simulink model "sim3d_14DoF_visualization"  (R2024b)
settings: Solver=VariableStepAuto  StartTime=0.0  StopTime=10.0  RelTol=1e-3
undefined symbols (not defined in the file or in its folder): sampleScene, simple_straight_unEven
libraries: sim3dlib x3, simulink x2, sim3dautolib x1
settings Model: Creator=fukuchi  LastModifiedBy=nobuakif

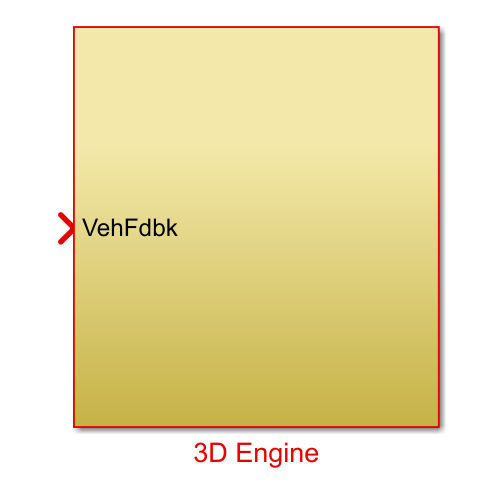
[thumbnail: Simulink's stored preview of the top-level diagram]
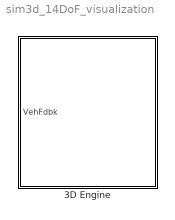
== system sim3d_14DoF_visualization ==
  3D Engine : Subsystem  VariantControl=engine3D==1

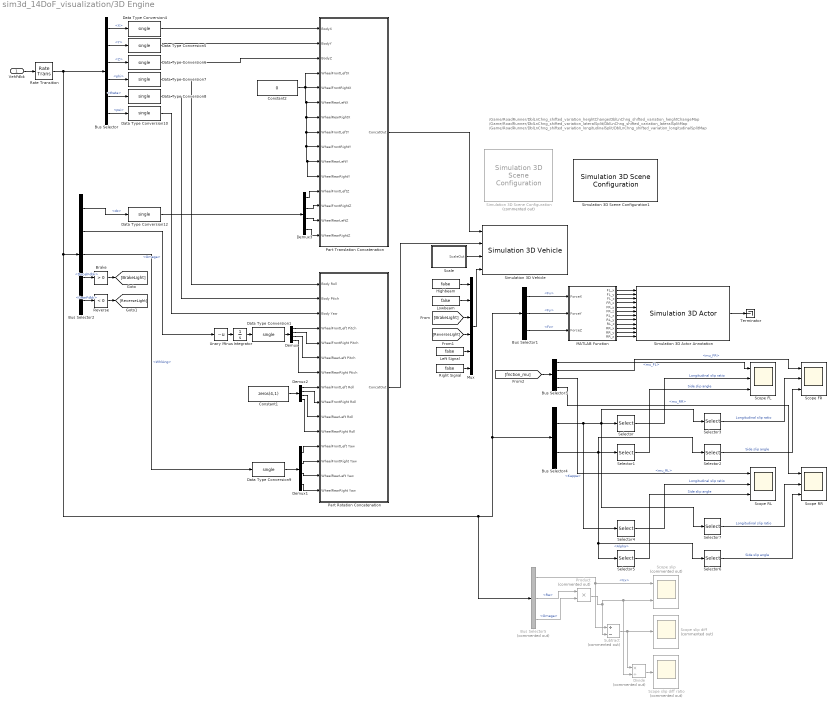
== system sim3d_14DoF_visualization/3D Engine ==
  note: /Game/RoadRunner/DblLnChng_shifted_variation_heightChange/DblLnChng_shifted_variation_heightChangeMap
      | /Game/RoadRunner/DblLnChng_shifted_variation_lateralSplit/DblLnChng_shifted_variation_lateralSplitMap
      | /Game/RoadRunner/DblLnChng_shifted_variation_longitudinalSplit/DblLnChng_shifted_variation_longitudinalSplitMap
  VehFdbk : Inport
  Brake : simulink/Logic and Bit Operations/Compare To Constant  relop=>  const=0  OutDataTypeStr=boolean  ZeroCross=off
  Bus Selector : BusSelector  OutputSignals=Body.InertFrm.Geom.Disp.X,Body.InertFrm.Geom.Disp.Y,Body.InertFrm.Geom.Disp.Z,Body.InertFrm.Cg.Ang.phi,Body.InertFrm.Cg.Ang.theta,Body.InertFrm.Cg.Ang.psi
  Bus Selector1 : BusSelector  OutputSignals=Wheels.TireFrame.Fx,Wheels.TireFrame.Fy,Wheels.TireFrame.Fz
  Bus Selector2 : BusSelector  OutputSignals=Wheels.TireFrame.dz,Wheels.TireFrame.Omega,Driveline.WhlAng,Driver.DecelFdbk,Driver.GearFdbk
  Bus Selector3 : BusSelector  OutputSignals=mu_FL,mu_FR,mu_RL,mu_RR
  Bus Selector4 : BusSelector  OutputSignals=Wheels.TireFrame.Kappa,Wheels.TireFrame.Alpha
  Bus Selector5 : BusSelector  Commented=on  OutputSignals=Wheels.TireFrame.Vx,Wheels.TireFrame.Re,Wheels.TireFrame.Omega
  Constant1 : Constant  Value=zeros(4,1)  OutDataTypeStr=single
  Constant2 : Constant  Value=0  OutDataTypeStr=single
  Data Type Conversion{1,4..10,12} (9 alike) : DataTypeConversion  OutDataTypeStr=single  SaturateOnIntegerOverflow=off  RndMeth=Floor
  Demux{,1..3} (4 alike) : Demux
  Divide : Product  Commented=on  Inputs=*/
  Highbeam : Constant  Value=false
  Integrator : Integrator  WrapState=on  WrappedStateUpperValue=2*pi  WrappedStateLowerValue=0  ZeroCross=off
  Left Signal : Constant  Value=false
  Lowbeam : Constant  Value=false
  MATLAB Function : MATLAB Function  TreatAsAtomicUnit=on
  Mux : Mux  Inputs=6
  Part Rotation Concatenation : Subsystem
  Part Translation Concatenation : Subsystem
  Product : Product  Commented=on
  Rate Transition : RateTransition  OutPortSampleTime=0.1
  Reverse : simulink/Logic and Bit Operations/Compare To Constant  relop=<  const=0  OutDataTypeStr=boolean  ZeroCross=off
  Right Signal : Constant  Value=false
  Scale : Subsystem
  Scope FL : Scope  NumInputPorts=3
  Scope FR : Scope  NumInputPorts=3
  Scope RL : Scope  NumInputPorts=3
  Scope RR : Scope  NumInputPorts=3
  Scope slip : Scope  Commented=on  NumInputPorts=2
  Scope slip diff : Scope  Commented=on
  Scope slip diff ratio : Scope  Commented=on
  Selector : Selector  InputPortWidth=4  IndexOptions=Index vector (dialog)  Indices=1  OutputSizes=1
  Selector1 : Selector  InputPortWidth=4  IndexOptions=Index vector (dialog)  Indices=1  OutputSizes=1
  Selector2 : Selector  InputPortWidth=4  IndexOptions=Index vector (dialog)  Indices=2  OutputSizes=1
  Selector3 : Selector  InputPortWidth=4  IndexOptions=Index vector (dialog)  Indices=2  OutputSizes=1
  Selector4 : Selector  InputPortWidth=4  IndexOptions=Index vector (dialog)  Indices=3  OutputSizes=1
  Selector5 : Selector  InputPortWidth=4  IndexOptions=Index vector (dialog)  Indices=3  OutputSizes=1
  Selector6 : Selector  InputPortWidth=4  IndexOptions=Index vector (dialog)  Indices=4  OutputSizes=1
  Selector7 : Selector  InputPortWidth=4  IndexOptions=Index vector (dialog)  Indices=4  OutputSizes=1
  Simulation 3D Actor Annotation : sim3dlib/Simulation 3D Actor  Priority=1  ActorName=Sim3dActor_annotation  ParentName=SimulinkVehicle1  Operation=Create at setup  InitScriptText=|  SampleTime=-1  Translation=single([0 0 0])  Rotation=single([0 0 0])  Scale=single([1 1 1])  InputsText=|  aMode=5  ActorTag=Sim3dActor_annotation  ActorType=Sim3dActor  ID=C
      InitScriptText=|
      | y_offset = 1; z_offset = 0.1;
      | fl_pos = [1.491, 1.713/2+y_offset, z_offset];
      | fr_pos = [1.491, -1.713/2-y_offset, z_offset];
      | rl_pos = [-1.592, 1.713/2+y_offset, z_offset];
      | rr_pos = [-1.592, -1.713/2-y_offset, z_offset];
      | 
      | arrowfl = sim3d.graphics.Arrow("ActorName", "FL_Z");
      | arrowfl.CoordinateSystem = "MATLAB";
      | arrowfl.Color = [0, 0, 1];
      | arrowfl.Rotation = [0, -pi/2, 0];
      | arrowfl.Scale = [1, 1, 1]*2;
      | World.add(arrowfl, Actor);
      | arrowfl.Translation = fl_pos;
      | 
      | arrowfl_x = sim3d.graphics.Arrow("ActorName", "FL_X");
      | arrowfl_x.CoordinateSystem = "MATLAB";
      | arrowfl_x.Color = [1, 0, 0];
      | arrowfl_x.Rotation = [0, 0, 0];
      | arrowfl_x.Scale = [1, 1, 1]*2;
      | World.add(arrowfl_x, Actor);
      | arrowfl_x.Translation = fl_pos;
      | 
      | arrowfl_y = sim3d.graphics.Arrow("ActorName", "FL_Y");
      | arrowfl_y.CoordinateSystem = "MATLAB";
      | arrowfl_y.Color = [0, 1, 0];
      | arrowfl_y.Rotation = [0, 0, pi/2];
      | arrowfl_y.Scale = [1, 1, 1]*2;
      | World.add(arrowfl_y, Actor);
      | arrowfl_y.Translation = fl_pos;
      | 
      | 
      | arrowfr = sim3d.graphics.Arrow("ActorName", "FR_Z");
      | arrowfr.CoordinateSystem = "MATLAB";
      | arrowfr.Color = [0, 0, 1];
      | arrowfr.Rotation = [0, -pi/2, 0];
      | arrowfr.Scale = [1, 1, 1] * 2;
      | World.add(arrowfr, Actor);
      | arrowfr.Translation = fr_pos;
      | 
      | arrowfr_x = sim3d.graphics.Arrow("ActorName", "FR_X");
      | arrowfr_x.CoordinateSystem = "MATLAB";
      | arrowfr_x.Color = [1, 0, 0];
      | arrowfr_x.Rotation = [0, 0, 0];
      | arrowfr_x.Scale = [1, 1, 1]*2;
      | World.add(arrowfr_x, Actor);
      | arrowfr_x.Translation = fr_pos;
      | 
      | arrowfr_y = sim3d.graphics.Arrow("ActorName", "FR_Y");
      | arrowfr_y.CoordinateSystem = "MATLAB";
      | arrowfr_y.Color = [0, 1, 0];
      | arrowfr_y.Rotation = [0, 0, pi/2];
      | arrowfr_y.Scale = [1, 1, 1]*2;
      | World.add(arrowfr_y, Actor);
      | arrowfr_y.Translation = fr_pos;
      | 
      | 
      | arrowrl = sim3d.graphics.Arrow("ActorName", "RL_Z");
      | arrowrl.CoordinateSystem = "MATLAB";
      | arrowrl.Color = [0, 0, 1];
      | arrowrl.Rotation = [0, -pi/2, 0];
      | arrowrl.Scale = [1, 1, 1] * 2;
      | World.add(arrowrl, Actor);
      | arrowrl.Translation = rl_pos;
      | 
      | arrowrl_x = sim3d.graphics.Arrow("ActorName", "RL_X");
      | arrowrl_x.CoordinateSystem = "MATLAB";
      | arrowrl_x.Color = [1, 0, 0];
      | arrowrl_x.Rotation = [0, 0, 0];
      | arrowrl_x.Scale = [1, 1, 1]*2;
      | World.add(arrowrl_x, Actor);
      | arrowrl_x.Translation = rl_pos;
      | 
      | arrowrl_y = sim3d.graphics.Arrow("ActorName", "RL_Y");
      | arrowrl_y.CoordinateSystem = "MATLAB";
      | arrowrl_y.Color = [0, 1, 0];
      | arrowrl_y.Rotation = [0, 0, pi/2];
      | arrowrl_y.Scale = [1, 1, 1]*2;
      | World.add(arrowrl_y, Actor);
      | arrowrl_y.Translation = rl_pos;
      | 
      | 
      | arrowrr = sim3d.graphics.Arrow("ActorName", "RR_Z");
      | arrowrr.CoordinateSystem = "MATLAB";
      | arrowrr.Color = [0, 0, 1];
      | arrowrr.Rotation = [0, -pi/2, 0];
      | arrowrr.Scale = [1, 1, 1]*2;
      | World.add(arrowrr, Actor);
      | arrowrr.Translation = rr_pos;
      | 
      | arrowrr_x = sim3d.graphics.Arrow("ActorName", "RR_X");
      | arrowrr_x.CoordinateSystem = "MATLAB";
      | arrowrr_x.Color = [1, 0, 0];
      | arrowrr_x.Rotation = [0, 0, 0];
      | arrowrr_x.Scale = [1, 1, 1]*2;
      | World.add(arrowrr_x, Actor);
      | arrowrr_x.Translation = rr_pos;
      | 
      | arrowrr_y = sim3d.graphics.Arrow("ActorName", "RR_Y");
      | arrowrr_y.CoordinateSystem = "MATLAB";
      | arrowrr_y.Color = [0, 1, 0];
      | arrowrr_y.Rotation = [0, 0, pi/2];
      | arrowrr_y.Scale = [1, 1, 1]*2;
      | World.add(arrowrr_y, Actor);
      | arrowrr_y.Translation = rr_pos;
      InputsText=|
      | FL_X.Scale
      | FL_Y.Scale
      | FL_Z.Scale
      | FR_X.Scale
      | FR_Y.Scale
      | FR_Z.Scale
      | RL_X.Scale
      | RL_Y.Scale
      | RL_Z.Scale
      | RR_X.Scale
      | RR_Y.Scale
      | RR_Z.Scale
  Simulation 3D Scene Configuration : sim3dlib/Simulation 3D Scene Configuration  Priority=0  Commented=on  ProjectFormat=RoadRunner  SceneDesc=Double lane change  ProjectName=D:\MATLAB\R2024b\toolbox\shared\sim3d_projects\automotive_project_windows\UE\WindowsNoEditor\VehicleSimulation.exe  ScenePath=/Game/RoadRunner/DblLnChng_shifted_variation_longitudinalSplit/DblLnChng_shifted_variation_longitudinalSplitMap  RoadRunnerProjectPath=sampleScene/simple_straight_unEven.fbx  UEProjPath=D:\ADT_UE4\R2024aGR\AutoVrtlEnv\AutoVrtlEnv.uproject  EnableOpenDRIVE=off  vehTagList={'Custom';'Scene Origin';'Sim3dActor_annotation';'SimulinkVehicle1'}  vehTag=Sim3dActor_annotation  FreeCameraInitialTranslation=[0, 0, 0]  FreeCameraDefaultInitialTranslation=[-6, 0, 2]  FreeCameraInitialRotation=[0, 0, 0]  FreeCameraDefaultInitialRotation=[0, -15, 0]  OpVisEn=off  Ts=0.1  EnableWindow=on  EnableRemoteAccess=off  EnableWeather=off  SunAzimuth=90  SunAltitude=40.0  EnableGeospatialSun=off  Latitude=0  Longitude=0  Date=2023-01-01  Time=10:30:00  GeoTimeZone=-5.0  SunDaylightSaving=off  wind=1  clouds=10  EnableVolumetricClouds=off  CloudCoverage=0  CloudAltitude=6  fog=0  rain=0  RaindropsEffect=off  SnowDensity=0  EnableGeospatial=off  UseTrueOrigin=off  OriginHeight=200  OriginLatitude=40.744652  OriginLongitude=-73.988864  MapStyle=Aerial  AdditionalAssetIDs=[]  UseAdvancedSunSky=off  SolarTime=11  TimeZone=-5  Day=21  Month=9  Year=2022  UseDaylightSavingTime=on  DSTStartDay=10  DSTStartMonth=3  DSTEndDay=3  DSTEndMonth=11  DSTSwitchHour=2  sensorTag=MainCamera1  sensorId=1  sensorName=MainCamera1  mountLoc=Origin  offsetFlag=off  tmountOffset=[0, 0, 0]  rmountOffset=[0, 0, 0]  HorizontalResolution=1280  VerticalResolution=720  HorizontalFOV=60  mountPoint=[0 0 0]  mountOrientation=[0 0 0]  aMode=2  ID=1  GeoTrigger=Inactive
      settings: LibrarySourceBlock=vehdynlibsim3dcore/Simulation 3D Scene Configuration
  Simulation 3D Scene Configuration1 : sim3dlib/Simulation 3D Scene Configuration  Priority=0  ProjectFormat=Default Scenes  SceneDesc=Empty scene  ProjectName=D:\MATLAB\R2024b\toolbox\shared\sim3d_projects\automotive_project_windows\UE\WindowsNoEditor\VehicleSimulation.exe  ScenePath=/Game/Maps/HwStrght  EnableOpenDRIVE=off  vehTagList={'Custom';'Scene Origin';'Sim3dActor_annotation';'SimulinkVehicle1'}  vehTag=SimulinkVehicle1  FreeCameraInitialTranslation=[0, 0, 0]  FreeCameraDefaultInitialTranslation=[-6, 0, 2]  FreeCameraInitialRotation=[0, 0, 0]  FreeCameraDefaultInitialRotation=[0, -15, 0]  OpVisEn=off  Ts=0.1  EnableWindow=on  EnableRemoteAccess=off  EnableWeather=off  SunAzimuth=90  SunAltitude=40.0  EnableGeospatialSun=off  Latitude=0  Longitude=0  Date=2023-01-01  Time=10:30:00  GeoTimeZone=-5.0  SunDaylightSaving=off  wind=1  clouds=10  EnableVolumetricClouds=off  CloudCoverage=0  CloudAltitude=6  fog=0  rain=0  RaindropsEffect=off  SnowDensity=0  EnableGeospatial=off  UseTrueOrigin=off  OriginHeight=200  OriginLatitude=40.744652  OriginLongitude=-73.988864  MapStyle=Aerial  AdditionalAssetIDs=[]  UseAdvancedSunSky=off  SolarTime=11  TimeZone=-5  Day=21  Month=9  Year=2022  UseDaylightSavingTime=on  DSTStartDay=10  DSTStartMonth=3  DSTEndDay=3  DSTEndMonth=11  DSTSwitchHour=2  sensorTag=MainCamera2  sensorId=2  sensorName=MainCamera2  mountLoc=Origin  offsetFlag=off  tmountOffset=[0, 0, 0]  rmountOffset=[0, 0, 0]  HorizontalResolution=1280  VerticalResolution=720  HorizontalFOV=60  mountPoint=[0 0 0]  mountOrientation=[0 0 0]  aMode=5  ID=2  GeoTrigger=Inactive
      settings: LibrarySourceBlock=sl3dlib/Simulation 3D/Environment/Simulation 3D Scene Configuration
  Simulation 3D Vehicle : sim3dautolib/Simulation 3D Vehicle  Priority=-1  PassVehMesh=Muscle car  MeshPath=/MathWorksSimulation/Vehicles/Muscle/Meshes/SK_MuscleCar.SK_MuscleCar  VehColor=Red  ActorName=SimulinkVehicle1  VehLightsControl=on  HeadlightColor=[ 1, 1, 1 ]  HighBeamIntensity=100000  LowBeamIntensity=60000  HighBeamConeAngle=1.22  LowBeamConeAngle=1.22  LeftHeadlightOrientation=[ 0, 0 ]  RightHeadlightOrientation=[ 0, 0 ]  BrakelightIntensity=500  ReverselightIntensity=500  SignallightIntensity=500  SignallightPeriod=1  SignalPulseWidth=50  Translation=zeros(5,3)  Rotation=zeros(5,3)  Scale=ones( 5, 3 )  SampleTime=-1  ActorType=SimulinkVehicle  ID=1  aMode=2  ActorTag=SimulinkVehicle1
  Subtract : Sum  Commented=on  Inputs=+-
  Terminator : Terminator
  Unary Minus : UnaryMinus
  wires:
  Unary Minus/1 -> Integrator/1
  Bus Selector2/1 -> Data Type Conversion12/1  "<dz>"
  Rate Transition/1 -> Bus Selector/1, Bus Selector2/1, Bus Selector5/1, Bus Selector1/1, Bus Selector4/1
  Scale/1(ScaleOut) -> Simulation 3D Vehicle/3
  Demux/4 -> Part Rotation Concatenation/7(WheelRearRight Ptich)
  Demux/3 -> Part Rotation Concatenation/6(WheelRearLeft Pitch)
  Demux/2 -> Part Rotation Concatenation/5(WheelFrontRight Pitch)
  Demux/1 -> Part Rotation Concatenation/4(WheelFrontLeft Pitch)
  Constant1/1 -> Demux2/1
  Bus Selector/4 -> Data Type Conversion7/1  "<phi>"
  Part Rotation Concatenation/1(ConcatOut) -> Simulation 3D Vehicle/2
  Part Translation Concatenation/1(ConcatOut) -> Simulation 3D Vehicle/1
  Data Type Conversion12/1 -> Demux3/1
  Demux3/4 -> Part Translation Concatenation/15(WheelRearRightZ)
  Demux3/3 -> Part Translation Concatenation/14(WheelRearLeftZ)
  Demux3/1 -> Part Translation Concatenation/12(WheelFrontLeftZ)
  Demux3/2 -> Part Translation Concatenation/13(WheelFrontRightZ)
  VehFdbk/1 -> Rate Transition/1
  Data Type Conversion6/1 -> Part Translation Concatenation/3(BodyZ)
  Demux1/4 -> Part Rotation Concatenation/15(WheelRearRight Yaw)
  Demux1/3 -> Part Rotation Concatenation/14(WheelRearLeft Yaw)
  Demux2/1 -> Part Rotation Concatenation/8(WheelFrontLeft Roll)
  Demux2/2 -> Part Rotation Concatenation/9(WheelFrontRight Roll)
  Demux2/3 -> Part Rotation Concatenation/10(WheelRearLeft Roll)
  Demux2/4 -> Part Rotation Concatenation/11(WheelRearRight Roll)
  Bus Selector2/3 -> Data Type Conversion9/1  "<WhlAng>"
  Bus Selector2/2 -> Unary Minus/1  "<Omega>"
  Data Type Conversion9/1 -> Demux1/1
  Demux1/1 -> Part Rotation Concatenation/12(WheelFrontLeft Yaw)
  Demux1/2 -> Part Rotation Concatenation/13(WheelFrontRight Yaw)
  Integrator/1 -> Data Type Conversion1/1
  Data Type Conversion1/1 -> Demux/1
  Data Type Conversion8/1 -> Part Rotation Concatenation/2(Body Ptich)
  Data Type Conversion5/1 -> Part Translation Concatenation/2(BodyY)
  Data Type Conversion10/1 -> Part Rotation Concatenation/3(Body Yaw)
  Constant2/1 -> Part Translation Concatenation/5(WheelFrontRightX), Part Translation Concatenation/6(WheelRearLeftX), Part Translation Concatenation/7(WheelRearRightX), Part Translation Concatenation/8(WheelFrontLeftY), Part Translation Concatenation/9(WheelFrontRightY), Part Translation Concatenation/10(WheelRearLeftY), Part Translation Concatenation/11(WheelRearRightY), Part Translation Concatenation/4(WheelFrontLeftX)
  Data Type Conversion4/1 -> Part Translation Concatenation/1(BodyX)
  Data Type Conversion7/1 -> Part Rotation Concatenation/1(Body Roll)
  Bus Selector/1 -> Data Type Conversion4/1  "<X>"
  Bus Selector/2 -> Data Type Conversion5/1  "<Y>"
  Bus Selector/3 -> Data Type Conversion6/1  "<Z>"
  Bus Selector/6 -> Data Type Conversion10/1  "<psi>"
  Bus Selector/5 -> Data Type Conversion8/1  "<theta>"
  [BrakeLight] -> Mux/3
  Mux/1 -> Simulation 3D Vehicle/4
  Brake/1 -> [BrakeLight]
  Highbeam/1 -> Mux/1
  Reverse/1 -> [ReverseLight]
  [ReverseLight] -> Mux/4
  Lowbeam/1 -> Mux/2
  Right Signal/1 -> Mux/6
  Left Signal/1 -> Mux/5
  Bus Selector2/4 -> Brake/1  "<DecelFdbk>"
  Bus Selector2/5 -> Reverse/1  "<GearFdbk>"
  Bus Selector1/1 -> MATLAB Function/1(ForceX)  "<Fx>"
  Bus Selector1/2 -> MATLAB Function/2(ForceY)  "<Fy>"
  Bus Selector1/3 -> MATLAB Function/3(ForceZ)  "<Fz>"
  MATLAB Function/1(FL_x) -> Simulation 3D Actor Annotation/1
  MATLAB Function/2(FL_y) -> Simulation 3D Actor Annotation/2
  MATLAB Function/3(FL_z) -> Simulation 3D Actor Annotation/3
  MATLAB Function/4(FR_x) -> Simulation 3D Actor Annotation/4
  MATLAB Function/5(FR_y) -> Simulation 3D Actor Annotation/5
  MATLAB Function/6(FR_z) -> Simulation 3D Actor Annotation/6
  MATLAB Function/7(RL_x) -> Simulation 3D Actor Annotation/7
  MATLAB Function/8(RL_y) -> Simulation 3D Actor Annotation/8
  MATLAB Function/9(RL_z) -> Simulation 3D Actor Annotation/9
  MATLAB Function/10(RR_x) -> Simulation 3D Actor Annotation/10
  MATLAB Function/11(RR_y) -> Simulation 3D Actor Annotation/11
  MATLAB Function/12(RR_z) -> Simulation 3D Actor Annotation/12
  [friction_mu] -> Bus Selector3/1
  Bus Selector3/1 -> Scope FL/1  "<mu_FL>"
  Selector/1 -> Scope FL/2  "Longitudinal slip ratio"
  Selector1/1 -> Scope FL/3  "Side slip angle"
  Bus Selector3/2 -> Scope FR/1  "<mu_FR>"
  Selector3/1 -> Scope FR/2  "Longitudinal slip ratio"
  Selector2/1 -> Scope FR/3  "Side slip angle"
  Selector6/1 -> Scope RR/3  "Side slip angle"
  Selector7/1 -> Scope RR/2  "Longitudinal slip ratio"
  Selector5/1 -> Scope RL/3  "Side slip angle"
  Selector4/1 -> Scope RL/2  "Longitudinal slip ratio"
  Bus Selector4/2 -> Selector5/1, Selector6/1, Selector2/1, Selector1/1  "<Alpha>"
  Bus Selector4/1 -> Selector4/1, Selector7/1, Selector3/1, Selector/1  "<Kappa>"
  Bus Selector3/3 -> Scope RL/1  "<mu_RL>"
  Bus Selector3/4 -> Scope RR/1  "<mu_RR>"
  Simulation 3D Actor Annotation/1 -> Terminator/1
  Bus Selector5/1 -> Subtract/1, Scope slip/1  "<Vx>"
  Bus Selector5/2 -> Product/1  "<Re>"
  Bus Selector5/3 -> Product/2  "<Omega>"
  Product/1 -> Subtract/2, Divide/2, Scope slip/2
  Subtract/1 -> Divide/1, Scope slip diff/1
  Divide/1 -> Scope slip diff ratio/1

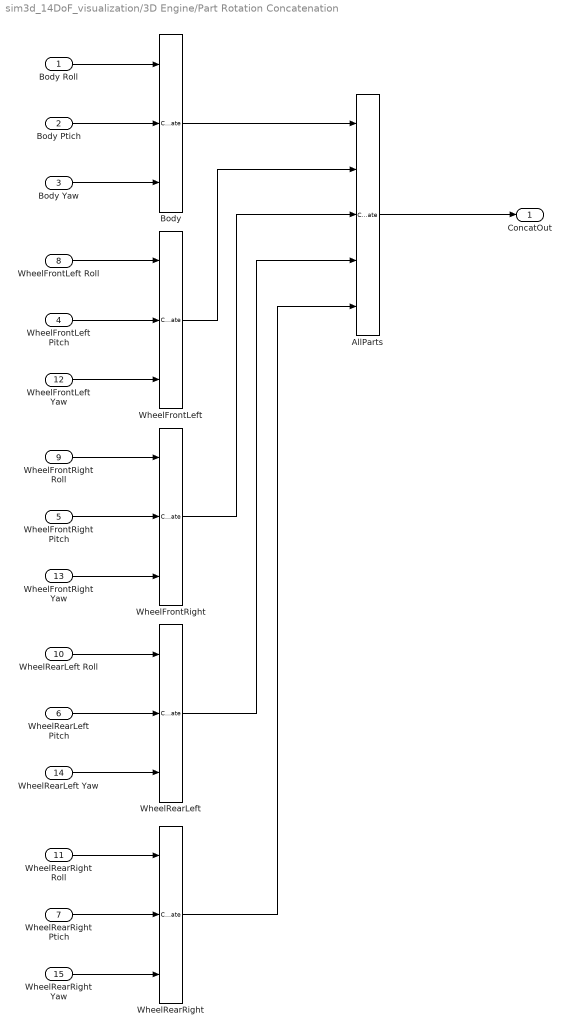
== system sim3d_14DoF_visualization/3D Engine/Part Rotation Concatenation ==
  Body Roll : Inport
  Body Ptich : Inport  Port=2
  Body Yaw : Inport  Port=3
  WheelFrontLeft Pitch : Inport  Port=4
  WheelFrontRight Pitch : Inport  Port=5
  WheelRearLeft Pitch : Inport  Port=6
  WheelRearRight Ptich : Inport  Port=7
  WheelFrontLeft Roll : Inport  Port=8
  WheelFrontRight Roll : Inport  Port=9
  WheelRearLeft Roll : Inport  Port=10
  WheelRearRight Roll : Inport  Port=11
  WheelFrontLeft Yaw : Inport  Port=12
  WheelFrontRight Yaw : Inport  Port=13
  WheelRearLeft Yaw : Inport  Port=14
  WheelRearRight Yaw : Inport  Port=15
  AllParts : Concatenate  NumInputs=5  Mode=Multidimensional array
  Body : Concatenate  NumInputs=3  Mode=Multidimensional array  ConcatenateDimension=2
  WheelFrontLeft : Concatenate  NumInputs=3  Mode=Multidimensional array  ConcatenateDimension=2
  WheelFrontRight : Concatenate  NumInputs=3  Mode=Multidimensional array  ConcatenateDimension=2
  WheelRearLeft : Concatenate  NumInputs=3  Mode=Multidimensional array  ConcatenateDimension=2
  WheelRearRight : Concatenate  NumInputs=3  Mode=Multidimensional array  ConcatenateDimension=2
  ConcatOut : Outport  VectorParamsAs1DForOutWhenUnconnected=off
  wires:
  Body Yaw/1 -> Body/3
  WheelFrontLeft Yaw/1 -> WheelFrontLeft/3
  WheelFrontLeft/1 -> AllParts/2
  Body/1 -> AllParts/1
  WheelRearLeft/1 -> AllParts/4
  WheelFrontRight/1 -> AllParts/3
  WheelRearRight Yaw/1 -> WheelRearRight/3
  WheelRearLeft Yaw/1 -> WheelRearLeft/3
  AllParts/1 -> ConcatOut/1
  WheelRearRight/1 -> AllParts/5
  WheelFrontRight Yaw/1 -> WheelFrontRight/3
  Body Roll/1 -> Body/1
  Body Ptich/1 -> Body/2
  WheelFrontLeft Pitch/1 -> WheelFrontLeft/2
  WheelFrontLeft Roll/1 -> WheelFrontLeft/1
  WheelFrontRight Roll/1 -> WheelFrontRight/1
  WheelFrontRight Pitch/1 -> WheelFrontRight/2
  WheelRearLeft Roll/1 -> WheelRearLeft/1
  WheelRearLeft Pitch/1 -> WheelRearLeft/2
  WheelRearRight Roll/1 -> WheelRearRight/1
  WheelRearRight Ptich/1 -> WheelRearRight/2

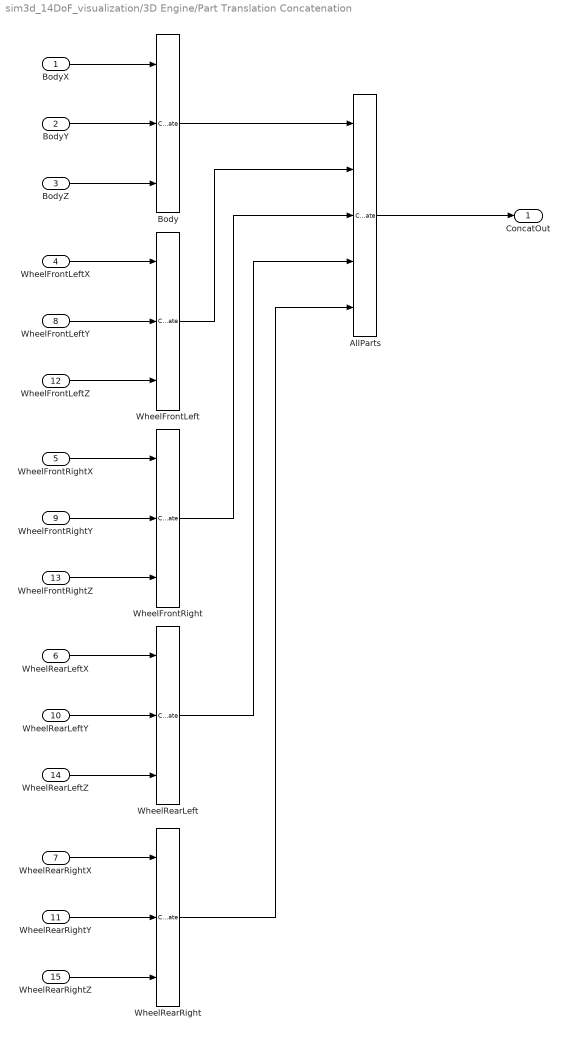
== system sim3d_14DoF_visualization/3D Engine/Part Translation Concatenation ==
  BodyX : Inport
  BodyY : Inport  Port=2
  BodyZ : Inport  Port=3
  WheelFrontLeftX : Inport  Port=4
  WheelFrontRightX : Inport  Port=5
  WheelRearLeftX : Inport  Port=6
  WheelRearRightX : Inport  Port=7
  WheelFrontLeftY : Inport  Port=8
  WheelFrontRightY : Inport  Port=9
  WheelRearLeftY : Inport  Port=10
  WheelRearRightY : Inport  Port=11
  WheelFrontLeftZ : Inport  Port=12
  WheelFrontRightZ : Inport  Port=13
  WheelRearLeftZ : Inport  Port=14
  WheelRearRightZ : Inport  Port=15
  AllParts : Concatenate  NumInputs=5  Mode=Multidimensional array
  Body : Concatenate  NumInputs=3  Mode=Multidimensional array  ConcatenateDimension=2
  WheelFrontLeft : Concatenate  NumInputs=3  Mode=Multidimensional array  ConcatenateDimension=2
  WheelFrontRight : Concatenate  NumInputs=3  Mode=Multidimensional array  ConcatenateDimension=2
  WheelRearLeft : Concatenate  NumInputs=3  Mode=Multidimensional array  ConcatenateDimension=2
  WheelRearRight : Concatenate  NumInputs=3  Mode=Multidimensional array  ConcatenateDimension=2
  ConcatOut : Outport  VectorParamsAs1DForOutWhenUnconnected=off
  wires:
  BodyX/1 -> Body/1
  BodyZ/1 -> Body/3
  WheelFrontLeftX/1 -> WheelFrontLeft/1
  WheelFrontLeftZ/1 -> WheelFrontLeft/3
  WheelFrontLeftY/1 -> WheelFrontLeft/2
  BodyY/1 -> Body/2
  WheelFrontLeft/1 -> AllParts/2
  WheelRearRightX/1 -> WheelRearRight/1
  Body/1 -> AllParts/1
  WheelRearLeft/1 -> AllParts/4
  WheelFrontRight/1 -> AllParts/3
  WheelRearRightZ/1 -> WheelRearRight/3
  WheelFrontRightY/1 -> WheelFrontRight/2
  WheelFrontRightX/1 -> WheelFrontRight/1
  WheelRearRightY/1 -> WheelRearRight/2
  WheelRearLeftZ/1 -> WheelRearLeft/3
  AllParts/1 -> ConcatOut/1
  WheelRearLeftY/1 -> WheelRearLeft/2
  WheelRearRight/1 -> AllParts/5
  WheelRearLeftX/1 -> WheelRearLeft/1
  WheelFrontRightZ/1 -> WheelFrontRight/3

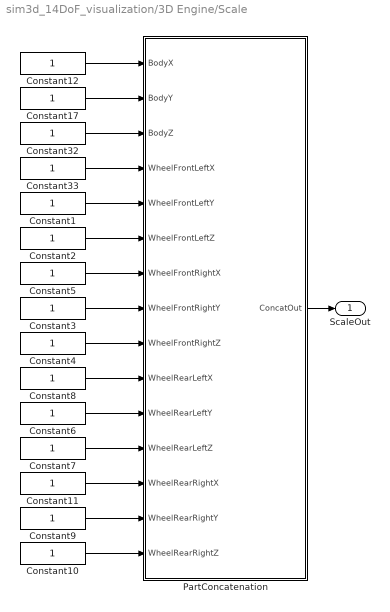
== system sim3d_14DoF_visualization/3D Engine/Scale ==
  Constant{1..12,17,32..33} (15 alike) : Constant  OutDataTypeStr=single
  PartConcatenation : Subsystem
  ScaleOut : Outport  VectorParamsAs1DForOutWhenUnconnected=off
  wires:
  Constant10/1 -> PartConcatenation/15(WheelRearRightZ)
  Constant9/1 -> PartConcatenation/14(WheelRearRightY)
  Constant11/1 -> PartConcatenation/13(WheelRearRightX)
  Constant7/1 -> PartConcatenation/12(WheelRearLeftZ)
  Constant6/1 -> PartConcatenation/11(WheelRearLeftY)
  Constant8/1 -> PartConcatenation/10(WheelRearLeftX)
  Constant4/1 -> PartConcatenation/9(WheelFrontRightZ)
  Constant3/1 -> PartConcatenation/8(WheelFrontRightY)
  Constant5/1 -> PartConcatenation/7(WheelFrontRightX)
  Constant2/1 -> PartConcatenation/6(WheelFrontLeftZ)
  Constant1/1 -> PartConcatenation/5(WheelFrontLeftY)
  Constant33/1 -> PartConcatenation/4(WheelFrontLeftX)
  Constant32/1 -> PartConcatenation/3(BodyZ)
  Constant17/1 -> PartConcatenation/2(BodyY)
  Constant12/1 -> PartConcatenation/1(BodyX)
  PartConcatenation/1(ConcatOut) -> ScaleOut/1

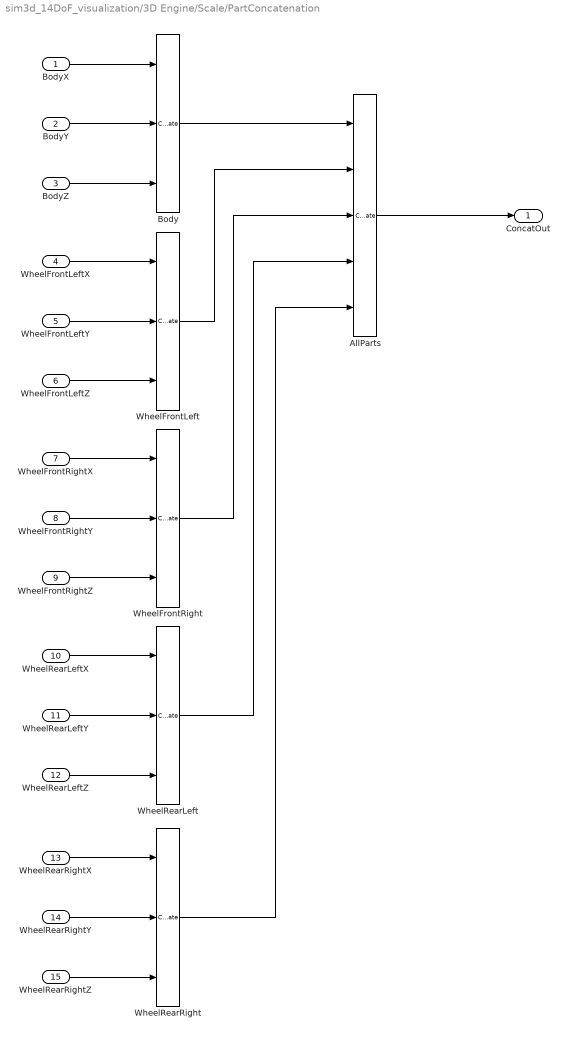
== system sim3d_14DoF_visualization/3D Engine/Scale/PartConcatenation ==
  BodyX : Inport
  BodyY : Inport  Port=2
  BodyZ : Inport  Port=3
  WheelFrontLeftX : Inport  Port=4
  WheelFrontLeftY : Inport  Port=5
  WheelFrontLeftZ : Inport  Port=6
  WheelFrontRightX : Inport  Port=7
  WheelFrontRightY : Inport  Port=8
  WheelFrontRightZ : Inport  Port=9
  WheelRearLeftX : Inport  Port=10
  WheelRearLeftY : Inport  Port=11
  WheelRearLeftZ : Inport  Port=12
  WheelRearRightX : Inport  Port=13
  WheelRearRightY : Inport  Port=14
  WheelRearRightZ : Inport  Port=15
  AllParts : Concatenate  NumInputs=5  Mode=Multidimensional array
  Body : Concatenate  NumInputs=3  Mode=Multidimensional array  ConcatenateDimension=2
  WheelFrontLeft : Concatenate  NumInputs=3  Mode=Multidimensional array  ConcatenateDimension=2
  WheelFrontRight : Concatenate  NumInputs=3  Mode=Multidimensional array  ConcatenateDimension=2
  WheelRearLeft : Concatenate  NumInputs=3  Mode=Multidimensional array  ConcatenateDimension=2
  WheelRearRight : Concatenate  NumInputs=3  Mode=Multidimensional array  ConcatenateDimension=2
  ConcatOut : Outport  VectorParamsAs1DForOutWhenUnconnected=off
  wires:
  BodyX/1 -> Body/1
  BodyZ/1 -> Body/3
  WheelFrontLeftX/1 -> WheelFrontLeft/1
  WheelFrontLeftZ/1 -> WheelFrontLeft/3
  WheelFrontLeftY/1 -> WheelFrontLeft/2
  BodyY/1 -> Body/2
  WheelFrontLeft/1 -> AllParts/2
  WheelRearRightX/1 -> WheelRearRight/1
  Body/1 -> AllParts/1
  WheelRearLeft/1 -> AllParts/4
  WheelFrontRight/1 -> AllParts/3
  WheelRearRightZ/1 -> WheelRearRight/3
  WheelFrontRightY/1 -> WheelFrontRight/2
  WheelFrontRightX/1 -> WheelFrontRight/1
  WheelRearRightY/1 -> WheelRearRight/2
  WheelRearLeftZ/1 -> WheelRearLeft/3
  AllParts/1 -> ConcatOut/1
  WheelRearLeftY/1 -> WheelRearLeft/2
  WheelRearRight/1 -> AllParts/5
  WheelRearLeftX/1 -> WheelRearLeft/1
  WheelFrontRightZ/1 -> WheelFrontRight/3

== matlab function sim3d_14DoF_visualization/3D Engine/MATLAB Function ==
  data: ForceX input; FL_x output; FL_y output; FL_z output; ForceY input; FR_x output; FR_y output; FR_z output; RL_x output; RL_y output; RL_z output; RR_x output; RR_y output; RR_z output; ForceZ input
function [FL_x, FL_y, FL_z, FR_x, FR_y, FR_z,...
    RL_x, RL_y, RL_z, RR_x, RR_y, RR_z] = fcn(ForceX, ForceY, ForceZ)

FL_x = [ForceX(1)/1000, 2, 2];
FL_y = [ForceY(1)/1000, 2, 2];
FL_z = [ForceZ(1)/1000, 2, 2];

FR_x = [ForceX(2)/1000, 2, 2];
FR_y = [ForceY(2)/1000, 2, 2];
FR_z = [ForceZ(2)/1000, 2, 2];

RL_x = [ForceX(3)/1000, 2, 2];
RL_y = [ForceY(3)/1000, 2, 2];
RL_z = [ForceZ(3)/1000, 2, 2];

RR_x = [ForceX(4)/1000, 2, 2];
RR_y = [ForceY(4)/1000, 2, 2];
RR_z = [ForceZ(4)/1000, 2, 2];
